simulink model "SystemArch"  (R2025a)
settings: Solver=VariableStepAuto  StartTime=0.0  StopTime=10.0  RelTol=1e-3
undefined symbols (not defined in the file): BMS, Camera, Digital, GPS, I2C, IMU, Trhemocouple, UART, UBS1, UBS2, USB1
(part 1 of 2)
settings Model: Creator=el2jo  LastModifiedBy=el2jo

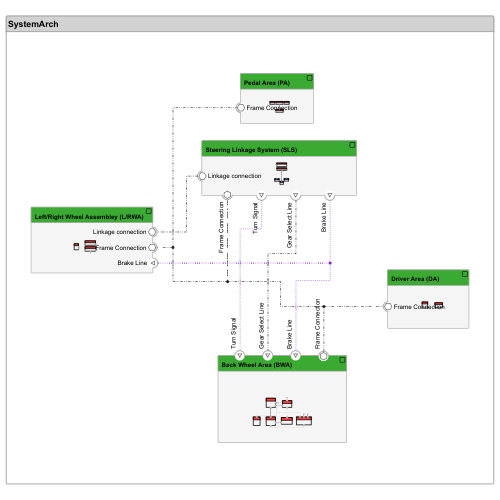
[thumbnail: Simulink's stored preview of the top-level diagram]
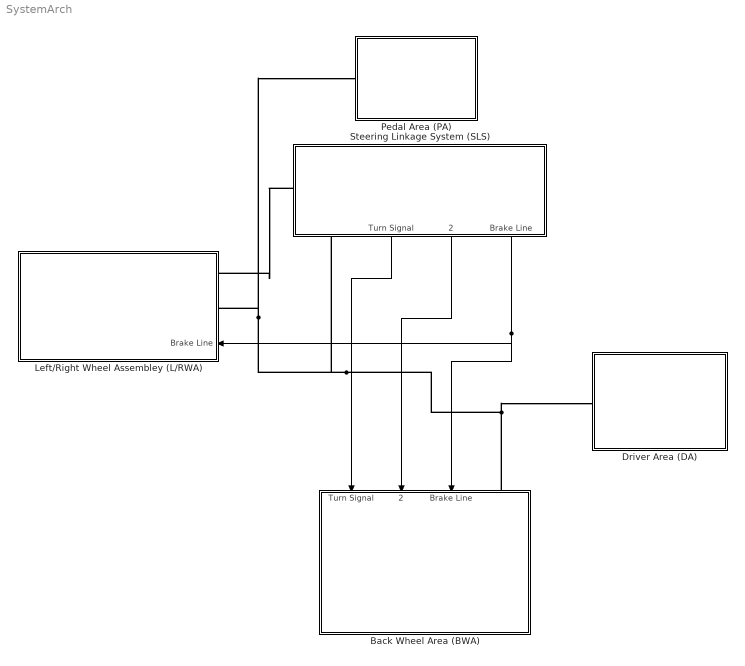
== system SystemArch ==
  "Back Wheel Area (BWA) " : Subsystem
      settings: PortSchema="{\"entries\":[{\"content\":{\"headerSize\":26,\"margin\":15,\"minimumSpacing\":25,\"sides\":[{\"content\":{},\"type\":\"ConnectorPlacement.EquallySpacedRectSide\",\"uuid\":\"b908bc96-20ac-41af-bd35-1dc4c5c5d227\"},{\"content\":{\"side\":\"RIGHT\"},\"type\":\"ConnectorPlacement.EquallySpacedRectSide\",\"uuid\":\"a58e5db6-c2cf-479b-8575-444173ed86e1\"},{\"content\":{\"connectorIds\":[\"In1\",\"In2\",\"In3\",\"LConn1\"],\"side\":\"TOP\"},\"type\":\"ConnectorPlacement.EquallySpacedRectSide\",\"uuid\":\"d8b1b400-2606-4583-b904-435fd1d8de03\"},{\"content\":{\"side\":\"BOTTOM\"},\"type\":\"ConnectorPlacement.EquallySpacedRectSide\",\"uuid\":\"75f2ceb6-2288-4f67-913e-11cbd02fad7a\"}]},\"type\":\"ConnectorPlacement.EquallySpacedConnector\",\"uuid\":\"bef962c1-e5c2-4b6f-9336-41c558e2844c\"}],\"packageUris\":[\"http://schema.mathworks.com/mf0/Connector/R2020b\"],\"version\":\"1.0\"}"
  Driver Area (DA) : Subsystem
      settings: PortSchema="{\"entries\":[{\"content\":{\"headerSize\":26,\"margin\":15,\"minimumSpacing\":25,\"sides\":[{\"content\":{\"connectorIds\":[\"RConn1\"]},\"type\":\"ConnectorPlacement.EquallySpacedRectSide\",\"uuid\":\"9a85c35e-563d-4a01-b414-04078d713158\"},{\"content\":{\"side\":\"RIGHT\"},\"type\":\"ConnectorPlacement.EquallySpacedRectSide\",\"uuid\":\"c9009d1a-5d28-4010-89bb-ea158d9a12da\"},{\"content\":{\"side\":\"TOP\"},\"type\":\"ConnectorPlacement.EquallySpacedRectSide\",\"uuid\":\"7ba794cc-3a18-4e87-89a3-ec47c4636e6e\"},{\"content\":{\"side\":\"BOTTOM\"},\"type\":\"ConnectorPlacement.EquallySpacedRectSide\",\"uuid\":\"f897e654-bc77-4131-98b6-05ede3c94ab0\"}]},\"type\":\"ConnectorPlacement.EquallySpacedConnector\",\"uuid\":\"a2b4ff38-2813-4eb8-955a-97f08d182cf4\"}],\"packageUris\":[\"http://schema.mathworks.com/mf0/Connector/R2020b\"],\"version\":\"1.0\"}"
  Left/Right Wheel Assembley (L/RWA) : Subsystem
      settings: PortSchema="{\"entries\":[{\"content\":{\"headerSize\":26,\"margin\":15,\"minimumSpacing\":25,\"sides\":[{\"content\":{},\"type\":\"ConnectorPlacement.EquallySpacedRectSide\",\"uuid\":\"9a85c35e-563d-4a01-b414-04078d713158\"},{\"content\":{\"connectorIds\":[\"RConn1\",\"RConn2\",\"In1\"],\"side\":\"RIGHT\"},\"type\":\"ConnectorPlacement.EquallySpacedRectSide\",\"uuid\":\"c9009d1a-5d28-4010-89bb-ea158d9a12da\"},{\"content\":{\"side\":\"TOP\"},\"type\":\"ConnectorPlacement.EquallySpacedRectSide\",\"uuid\":\"7ba794cc-3a18-4e87-89a3-ec47c4636e6e\"},{\"content\":{\"side\":\"BOTTOM\"},\"type\":\"ConnectorPlacement.EquallySpacedRectSide\",\"uuid\":\"b9e3f91c-afcc-4ee7-a70b-ea22bbb4204d\"}]},\"type\":\"ConnectorPlacement.EquallySpacedConnector\",\"uuid\":\"a2b4ff38-2813-4eb8-955a-97f08d182cf4\"}],\"packageUris\":[\"http://schema.mathworks.com/mf0/Connector/R2020b\"],\"version\":\"1.0\"}"
  Pedal Area (PA) : Subsystem
      settings: PortSchema="{\"entries\":[{\"content\":{\"headerSize\":26,\"margin\":15,\"minimumSpacing\":25,\"sides\":[{\"content\":{\"connectorIds\":[\"RConn1\"]},\"type\":\"ConnectorPlacement.EquallySpacedRectSide\",\"uuid\":\"9a85c35e-563d-4a01-b414-04078d713158\"},{\"content\":{\"side\":\"RIGHT\"},\"type\":\"ConnectorPlacement.EquallySpacedRectSide\",\"uuid\":\"c9009d1a-5d28-4010-89bb-ea158d9a12da\"},{\"content\":{\"side\":\"TOP\"},\"type\":\"ConnectorPlacement.EquallySpacedRectSide\",\"uuid\":\"7ba794cc-3a18-4e87-89a3-ec47c4636e6e\"},{\"content\":{\"side\":\"BOTTOM\"},\"type\":\"ConnectorPlacement.EquallySpacedRectSide\",\"uuid\":\"443625ad-4830-4e83-8594-463a9c2e837b\"}]},\"type\":\"ConnectorPlacement.EquallySpacedConnector\",\"uuid\":\"a2b4ff38-2813-4eb8-955a-97f08d182cf4\"}],\"packageUris\":[\"http://schema.mathworks.com/mf0/Connector/R2020b\"],\"version\":\"1.0\"}"
  Steering Linkage System (SLS) : Subsystem
      settings: PortSchema="{\"entries\":[{\"content\":{\"headerSize\":26,\"margin\":15,\"minimumSpacing\":25,\"sides\":[{\"content\":{\"connectorIds\":[\"RConn1\"]},\"type\":\"ConnectorPlacement.EquallySpacedRectSide\",\"uuid\":\"9a85c35e-563d-4a01-b414-04078d713158\"},{\"content\":{\"side\":\"RIGHT\"},\"type\":\"ConnectorPlacement.EquallySpacedRectSide\",\"uuid\":\"c9009d1a-5d28-4010-89bb-ea158d9a12da\"},{\"content\":{\"side\":\"TOP\"},\"type\":\"ConnectorPlacement.EquallySpacedRectSide\",\"uuid\":\"7ba794cc-3a18-4e87-89a3-ec47c4636e6e\"},{\"content\":{\"connectorIds\":[\"RConn2\",\"Out1\",\"Out2\",\"Out3\"],\"side\":\"BOTTOM\"},\"type\":\"ConnectorPlacement.EquallySpacedRectSide\",\"uuid\":\"ee526e7b-a27e-4264-aa86-39ffcd82e9f9\"}]},\"type\":\"ConnectorPlacement.EquallySpacedConnector\",\"uuid\":\"a2b4ff38-2813-4eb8-955a-97f08d182cf4\"}],\"packageUris\":[\"http://schema.mathworks.com/mf0/Connector/R2020b\"],\"version\":\"1.0\"}"
  wires:
  Steering Linkage System (SLS)/1(Turn Signal) -> "Back Wheel Area (BWA) "/1(Turn Signal)
  Steering Linkage System (SLS)/2(Gear Select Line) -> "Back Wheel Area (BWA) "/2(Gear Select Line)
  Steering Linkage System (SLS)/3(Brake Line) -> Left/Right Wheel Assembley (L/RWA)/1(Brake Line), "Back Wheel Area (BWA) "/3(Brake Line)
  connections:
  "Back Wheel Area (BWA) "/LConn1 -- Steering Linkage System (SLS)/RConn2 -- Pedal Area (PA)/RConn1 -- Left/Right Wheel Assembley (L/RWA)/RConn2 -- Driver Area (DA)/RConn1
  Steering Linkage System (SLS)/RConn1 -- Left/Right Wheel Assembley (L/RWA)/RConn1

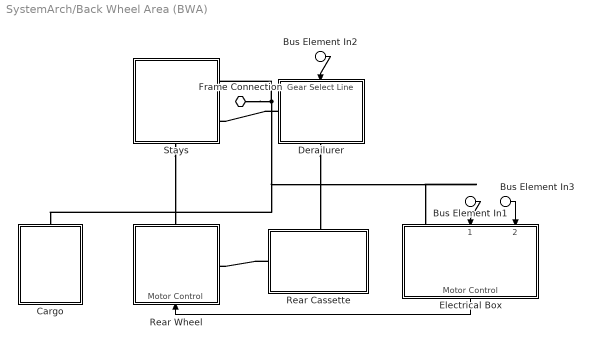
== system SystemArch/Back Wheel Area (BWA)  ==
  Bus Element In1 : Inport  PortName=Turn Signal
  Bus Element In2 : Inport  Port=2  PortName=Gear Select Line
  Bus Element In3 : Inport  Port=3  PortName=Brake Line
  "  Rear Cassette" : Subsystem
      settings: PortSchema="{\"entries\":[{\"content\":{\"headerSize\":26,\"margin\":15,\"minimumSpacing\":25,\"sides\":[{\"content\":{\"connectorIds\":[\"LConn2\"]},\"type\":\"ConnectorPlacement.EquallySpacedRectSide\",\"uuid\":\"9a85c35e-563d-4a01-b414-04078d713158\"},{\"content\":{\"side\":\"RIGHT\"},\"type\":\"ConnectorPlacement.EquallySpacedRectSide\",\"uuid\":\"c9009d1a-5d28-4010-89bb-ea158d9a12da\"},{\"content\":{\"connectorIds\":[\"LConn1\"],\"side\":\"TOP\"},\"type\":\"ConnectorPlacement.EquallySpacedRectSide\",\"uuid\":\"7ba794cc-3a18-4e87-89a3-ec47c4636e6e\"}]},\"type\":\"ConnectorPlacement.EquallySpacedConnector\",\"uuid\":\"a2b4ff38-2813-4eb8-955a-97f08d182cf4\"}],\"packageUris\":[\"http://schema.mathworks.com/mf0/Connector/R2020b\"],\"version\":\"1.0\"}"
  Cargo : Subsystem
      settings: PortSchema="{\"entries\":[{\"content\":{\"headerSize\":26,\"margin\":15,\"minimumSpacing\":25,\"sides\":[{\"content\":{},\"type\":\"ConnectorPlacement.EquallySpacedRectSide\",\"uuid\":\"9a85c35e-563d-4a01-b414-04078d713158\"},{\"content\":{\"side\":\"RIGHT\"},\"type\":\"ConnectorPlacement.EquallySpacedRectSide\",\"uuid\":\"c9009d1a-5d28-4010-89bb-ea158d9a12da\"},{\"content\":{\"connectorIds\":[\"LConn1\"],\"side\":\"TOP\"},\"type\":\"ConnectorPlacement.EquallySpacedRectSide\",\"uuid\":\"7ba794cc-3a18-4e87-89a3-ec47c4636e6e\"}]},\"type\":\"ConnectorPlacement.EquallySpacedConnector\",\"uuid\":\"a2b4ff38-2813-4eb8-955a-97f08d182cf4\"}],\"packageUris\":[\"http://schema.mathworks.com/mf0/Connector/R2020b\"],\"version\":\"1.0\"}"
  Derailurer : Subsystem
      settings: PortSchema="{\"entries\":[{\"content\":{\"headerSize\":26,\"margin\":15,\"minimumSpacing\":25,\"sides\":[{\"content\":{\"connectorIds\":[\"LConn1\"]},\"type\":\"ConnectorPlacement.EquallySpacedRectSide\",\"uuid\":\"9a85c35e-563d-4a01-b414-04078d713158\"},{\"content\":{\"side\":\"RIGHT\"},\"type\":\"ConnectorPlacement.EquallySpacedRectSide\",\"uuid\":\"c9009d1a-5d28-4010-89bb-ea158d9a12da\"},{\"content\":{\"connectorIds\":[\"In1\"],\"side\":\"TOP\"},\"type\":\"ConnectorPlacement.EquallySpacedRectSide\",\"uuid\":\"7ba794cc-3a18-4e87-89a3-ec47c4636e6e\"},{\"content\":{\"connectorIds\":[\"RConn1\"],\"side\":\"BOTTOM\"},\"type\":\"ConnectorPlacement.EquallySpacedRectSide\",\"uuid\":\"612b2382-3768-40cf-8c67-0c3e27c64c6d\"}]},\"type\":\"ConnectorPlacement.EquallySpacedConnector\",\"uuid\":\"a2b4ff38-2813-4eb8-955a-97f08d182cf4\"}],\"packageUris\":[\"http://schema.mathworks.com/mf0/Connector/R2020b\"],\"version\":\"1.0\"}"
  Electrical Box : Subsystem
      settings: PortSchema="{\"entries\":[{\"content\":{\"headerSize\":26,\"margin\":15,\"minimumSpacing\":25,\"sides\":[{\"content\":{},\"type\":\"ConnectorPlacement.EquallySpacedRectSide\",\"uuid\":\"b908bc96-20ac-41af-bd35-1dc4c5c5d227\"},{\"content\":{\"side\":\"RIGHT\"},\"type\":\"ConnectorPlacement.EquallySpacedRectSide\",\"uuid\":\"a58e5db6-c2cf-479b-8575-444173ed86e1\"},{\"content\":{\"connectorIds\":[\"LConn1\",\"In1\",\"In2\"],\"side\":\"TOP\"},\"type\":\"ConnectorPlacement.EquallySpacedRectSide\",\"uuid\":\"d8b1b400-2606-4583-b904-435fd1d8de03\"},{\"content\":{\"connectorIds\":[\"Out1\"],\"side\":\"BOTTOM\"},\"type\":\"ConnectorPlacement.EquallySpacedRectSide\",\"uuid\":\"a50bf375-f8fa-400b-8497-e942a7ca09d1\"}]},\"type\":\"ConnectorPlacement.EquallySpacedConnector\",\"uuid\":\"bef962c1-e5c2-4b6f-9336-41c558e2844c\"}],\"packageUris\":[\"http://schema.mathworks.com/mf0/Connector/R2020b\"],\"version\":\"1.0\"}"
  Rear Wheel : Subsystem
      settings: PortSchema="{\"entries\":[{\"content\":{\"headerSize\":26,\"margin\":15,\"minimumSpacing\":25,\"sides\":[{\"content\":{},\"type\":\"ConnectorPlacement.EquallySpacedRectSide\",\"uuid\":\"9a85c35e-563d-4a01-b414-04078d713158\"},{\"content\":{\"connectorIds\":[\"RConn1\"],\"side\":\"RIGHT\"},\"type\":\"ConnectorPlacement.EquallySpacedRectSide\",\"uuid\":\"c9009d1a-5d28-4010-89bb-ea158d9a12da\"},{\"content\":{\"connectorIds\":[\"LConn1\"],\"side\":\"TOP\"},\"type\":\"ConnectorPlacement.EquallySpacedRectSide\",\"uuid\":\"7ba794cc-3a18-4e87-89a3-ec47c4636e6e\"},{\"content\":{\"connectorIds\":[\"In1\"],\"side\":\"BOTTOM\"},\"type\":\"ConnectorPlacement.EquallySpacedRectSide\",\"uuid\":\"790efda8-cec0-4a27-8622-bef3d471aaff\"}]},\"type\":\"ConnectorPlacement.EquallySpacedConnector\",\"uuid\":\"a2b4ff38-2813-4eb8-955a-97f08d182cf4\"}],\"packageUris\":[\"http://schema.mathworks.com/mf0/Connector/R2020b\"],\"version\":\"1.0\"}"
  Stays : Subsystem
      settings: PortSchema="{\"entries\":[{\"content\":{\"headerSize\":26,\"margin\":15,\"minimumSpacing\":25,\"sides\":[{\"content\":{},\"type\":\"ConnectorPlacement.EquallySpacedRectSide\",\"uuid\":\"9a85c35e-563d-4a01-b414-04078d713158\"},{\"content\":{\"connectorIds\":[\"LConn1\",\"RConn1\"],\"side\":\"RIGHT\"},\"type\":\"ConnectorPlacement.EquallySpacedRectSide\",\"uuid\":\"c9009d1a-5d28-4010-89bb-ea158d9a12da\"},{\"content\":{\"side\":\"TOP\"},\"type\":\"ConnectorPlacement.EquallySpacedRectSide\",\"uuid\":\"7ba794cc-3a18-4e87-89a3-ec47c4636e6e\"},{\"content\":{\"connectorIds\":[\"RConn2\"],\"side\":\"BOTTOM\"},\"type\":\"ConnectorPlacement.EquallySpacedRectSide\",\"uuid\":\"d8ca6e35-2892-477f-b035-8e0ebcbafa05\"}]},\"type\":\"ConnectorPlacement.EquallySpacedConnector\",\"uuid\":\"a2b4ff38-2813-4eb8-955a-97f08d182cf4\"}],\"packageUris\":[\"http://schema.mathworks.com/mf0/Connector/R2020b\"],\"version\":\"1.0\"}"
  Frame Connection : PMIOPort  Side=Left
  wires:
  Electrical Box/1(Motor Control) -> Rear Wheel/1(Motor Control)
  Bus Element In2/1 -> Derailurer/1(Gear Select Line)
  Bus Element In1/1 -> Electrical Box/1(Turn Signal)
  Bus Element In3/1 -> Electrical Box/2(Brake Line)
  connections:
  Stays/RConn2 -- Rear Wheel/LConn1
  Frame Connection/RConn1 -- Cargo/LConn1 -- Electrical Box/LConn1 -- Stays/LConn1
  "  Rear Cassette"/LConn2 -- Rear Wheel/RConn1
  Derailurer/LConn1 -- Stays/RConn1
  Derailurer/RConn1 -- "  Rear Cassette"/LConn1

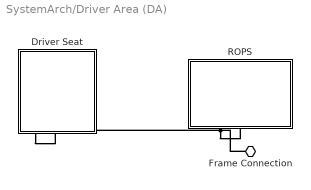
== system SystemArch/Driver Area (DA) ==
  Driver Seat : Subsystem
      settings: PortSchema="{\"entries\":[{\"content\":{\"headerSize\":26,\"margin\":15,\"minimumSpacing\":25,\"sides\":[{\"content\":{},\"type\":\"ConnectorPlacement.EquallySpacedRectSide\",\"uuid\":\"9a85c35e-563d-4a01-b414-04078d713158\"},{\"content\":{\"side\":\"RIGHT\"},\"type\":\"ConnectorPlacement.EquallySpacedRectSide\",\"uuid\":\"c9009d1a-5d28-4010-89bb-ea158d9a12da\"},{\"content\":{\"side\":\"TOP\"},\"type\":\"ConnectorPlacement.EquallySpacedRectSide\",\"uuid\":\"7ba794cc-3a18-4e87-89a3-ec47c4636e6e\"},{\"content\":{\"connectorIds\":[\"RConn1\"],\"side\":\"BOTTOM\"},\"type\":\"ConnectorPlacement.EquallySpacedRectSide\",\"uuid\":\"08e026bb-01c5-465b-bb8c-e734b87ff441\"}]},\"type\":\"ConnectorPlacement.EquallySpacedConnector\",\"uuid\":\"a2b4ff38-2813-4eb8-955a-97f08d182cf4\"}],\"packageUris\":[\"http://schema.mathworks.com/mf0/Connector/R2020b\"],\"version\":\"1.0\"}"
  ROPS : Subsystem
      settings: PortSchema="{\"entries\":[{\"content\":{\"headerSize\":26,\"margin\":15,\"minimumSpacing\":25,\"sides\":[{\"content\":{},\"type\":\"ConnectorPlacement.EquallySpacedRectSide\",\"uuid\":\"9a85c35e-563d-4a01-b414-04078d713158\"},{\"content\":{\"side\":\"RIGHT\"},\"type\":\"ConnectorPlacement.EquallySpacedRectSide\",\"uuid\":\"c9009d1a-5d28-4010-89bb-ea158d9a12da\"},{\"content\":{\"side\":\"TOP\"},\"type\":\"ConnectorPlacement.EquallySpacedRectSide\",\"uuid\":\"7ba794cc-3a18-4e87-89a3-ec47c4636e6e\"},{\"content\":{\"connectorIds\":[\"RConn1\"],\"side\":\"BOTTOM\"},\"type\":\"ConnectorPlacement.EquallySpacedRectSide\",\"uuid\":\"f6e8be95-bb09-4692-bbab-764924998958\"}]},\"type\":\"ConnectorPlacement.EquallySpacedConnector\",\"uuid\":\"a2b4ff38-2813-4eb8-955a-97f08d182cf4\"}],\"packageUris\":[\"http://schema.mathworks.com/mf0/Connector/R2020b\"],\"version\":\"1.0\"}"
  Frame Connection : PMIOPort  Side=Right
  connections:
  Frame Connection/RConn1 -- Driver Seat/RConn1 -- ROPS/RConn1

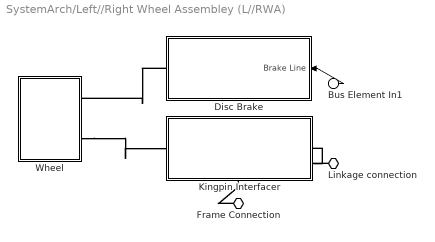
== system SystemArch/Left//Right Wheel Assembley (L//RWA) ==
  Bus Element In1 : Inport  PortName=Brake Line
  Disc Brake : Subsystem
      settings: PortSchema="{\"entries\":[{\"content\":{\"headerSize\":26,\"margin\":15,\"minimumSpacing\":25,\"sides\":[{\"content\":{\"connectorIds\":[\"LConn1\"]},\"type\":\"ConnectorPlacement.EquallySpacedRectSide\",\"uuid\":\"9a85c35e-563d-4a01-b414-04078d713158\"},{\"content\":{\"connectorIds\":[\"In1\"],\"side\":\"RIGHT\"},\"type\":\"ConnectorPlacement.EquallySpacedRectSide\",\"uuid\":\"c9009d1a-5d28-4010-89bb-ea158d9a12da\"},{\"content\":{\"side\":\"TOP\"},\"type\":\"ConnectorPlacement.EquallySpacedRectSide\",\"uuid\":\"7ba794cc-3a18-4e87-89a3-ec47c4636e6e\"}]},\"type\":\"ConnectorPlacement.EquallySpacedConnector\",\"uuid\":\"a2b4ff38-2813-4eb8-955a-97f08d182cf4\"}],\"packageUris\":[\"http://schema.mathworks.com/mf0/Connector/R2020b\"],\"version\":\"1.0\"}"
  Kingpin Interfacer : Subsystem
      settings: PortSchema="{\"entries\":[{\"content\":{\"headerSize\":26,\"margin\":15,\"minimumSpacing\":25,\"sides\":[{\"content\":{\"connectorIds\":[\"RConn3\"]},\"type\":\"ConnectorPlacement.EquallySpacedRectSide\",\"uuid\":\"9a85c35e-563d-4a01-b414-04078d713158\"},{\"content\":{\"connectorIds\":[\"RConn2\"],\"side\":\"RIGHT\"},\"type\":\"ConnectorPlacement.EquallySpacedRectSide\",\"uuid\":\"c9009d1a-5d28-4010-89bb-ea158d9a12da\"},{\"content\":{\"side\":\"TOP\"},\"type\":\"ConnectorPlacement.EquallySpacedRectSide\",\"uuid\":\"7ba794cc-3a18-4e87-89a3-ec47c4636e6e\"},{\"content\":{\"connectorIds\":[\"RConn1\"],\"side\":\"BOTTOM\"},\"type\":\"ConnectorPlacement.EquallySpacedRectSide\",\"uuid\":\"1146683b-fd7d-4bc2-bfc7-5416f68f0a28\"}]},\"type\":\"ConnectorPlacement.EquallySpacedConnector\",\"uuid\":\"a2b4ff38-2813-4eb8-955a-97f08d182cf4\"}],\"packageUris\":[\"http://schema.mathworks.com/mf0/Connector/R2020b\"],\"version\":\"1.0\"}"
  Wheel : Subsystem
      settings: PortSchema="{\"entries\":[{\"content\":{\"headerSize\":26,\"margin\":15,\"minimumSpacing\":25,\"sides\":[{\"content\":{},\"type\":\"ConnectorPlacement.EquallySpacedRectSide\",\"uuid\":\"9a85c35e-563d-4a01-b414-04078d713158\"},{\"content\":{\"connectorIds\":[\"RConn1\",\"RConn2\"],\"side\":\"RIGHT\"},\"type\":\"ConnectorPlacement.EquallySpacedRectSide\",\"uuid\":\"c9009d1a-5d28-4010-89bb-ea158d9a12da\"},{\"content\":{\"side\":\"TOP\"},\"type\":\"ConnectorPlacement.EquallySpacedRectSide\",\"uuid\":\"7ba794cc-3a18-4e87-89a3-ec47c4636e6e\"},{\"content\":{\"side\":\"BOTTOM\"},\"type\":\"ConnectorPlacement.EquallySpacedRectSide\",\"uuid\":\"b840c23f-69d1-4217-b707-91eb7d19865c\"}]},\"type\":\"ConnectorPlacement.EquallySpacedConnector\",\"uuid\":\"a2b4ff38-2813-4eb8-955a-97f08d182cf4\"}],\"packageUris\":[\"http://schema.mathworks.com/mf0/Connector/R2020b\"],\"version\":\"1.0\"}"
  Linkage connection : PMIOPort  Side=Right
  Frame Connection : PMIOPort  Port=2  Side=Right
  wires:
  Bus Element In1/1 -> Disc Brake/1(Brake Line)
  connections:
  Wheel/RConn2 -- Kingpin Interfacer/RConn3
  Disc Brake/LConn1 -- Wheel/RConn1
  Linkage connection/RConn1 -- Kingpin Interfacer/RConn2
  Frame Connection/RConn1 -- Kingpin Interfacer/RConn1

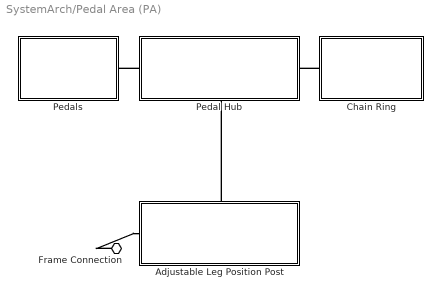
== system SystemArch/Pedal Area (PA) ==
  Adjustable Leg Position Post : Subsystem
      settings: PortSchema="{\"entries\":[{\"content\":{\"headerSize\":26,\"margin\":15,\"minimumSpacing\":25,\"sides\":[{\"content\":{\"connectorIds\":[\"LConn1\"]},\"type\":\"ConnectorPlacement.EquallySpacedRectSide\",\"uuid\":\"9a85c35e-563d-4a01-b414-04078d713158\"},{\"content\":{\"side\":\"RIGHT\"},\"type\":\"ConnectorPlacement.EquallySpacedRectSide\",\"uuid\":\"c9009d1a-5d28-4010-89bb-ea158d9a12da\"},{\"content\":{\"connectorIds\":[\"LConn2\"],\"side\":\"TOP\"},\"type\":\"ConnectorPlacement.EquallySpacedRectSide\",\"uuid\":\"7ba794cc-3a18-4e87-89a3-ec47c4636e6e\"}]},\"type\":\"ConnectorPlacement.EquallySpacedConnector\",\"uuid\":\"a2b4ff38-2813-4eb8-955a-97f08d182cf4\"}],\"packageUris\":[\"http://schema.mathworks.com/mf0/Connector/R2020b\"],\"version\":\"1.0\"}"
  Chain Ring : Subsystem
      settings: PortSchema="{\"entries\":[{\"content\":{\"headerSize\":26,\"margin\":15,\"minimumSpacing\":25,\"sides\":[{\"content\":{\"connectorIds\":[\"LConn1\"]},\"type\":\"ConnectorPlacement.EquallySpacedRectSide\",\"uuid\":\"9a85c35e-563d-4a01-b414-04078d713158\"},{\"content\":{\"side\":\"RIGHT\"},\"type\":\"ConnectorPlacement.EquallySpacedRectSide\",\"uuid\":\"c9009d1a-5d28-4010-89bb-ea158d9a12da\"},{\"content\":{\"side\":\"TOP\"},\"type\":\"ConnectorPlacement.EquallySpacedRectSide\",\"uuid\":\"7ba794cc-3a18-4e87-89a3-ec47c4636e6e\"}]},\"type\":\"ConnectorPlacement.EquallySpacedConnector\",\"uuid\":\"a2b4ff38-2813-4eb8-955a-97f08d182cf4\"}],\"packageUris\":[\"http://schema.mathworks.com/mf0/Connector/R2020b\"],\"version\":\"1.0\"}"
  Pedal Hub : Subsystem
      settings: PortSchema="{\"entries\":[{\"content\":{\"headerSize\":26,\"margin\":15,\"minimumSpacing\":25,\"sides\":[{\"content\":{\"connectorIds\":[\"LConn1\"]},\"type\":\"ConnectorPlacement.EquallySpacedRectSide\",\"uuid\":\"9a85c35e-563d-4a01-b414-04078d713158\"},{\"content\":{\"connectorIds\":[\"RConn1\"],\"side\":\"RIGHT\"},\"type\":\"ConnectorPlacement.EquallySpacedRectSide\",\"uuid\":\"c9009d1a-5d28-4010-89bb-ea158d9a12da\"},{\"content\":{\"side\":\"TOP\"},\"type\":\"ConnectorPlacement.EquallySpacedRectSide\",\"uuid\":\"7ba794cc-3a18-4e87-89a3-ec47c4636e6e\"},{\"content\":{\"connectorIds\":[\"RConn2\"],\"side\":\"BOTTOM\"},\"type\":\"ConnectorPlacement.EquallySpacedRectSide\",\"uuid\":\"d446abce-ebed-4a7d-b07b-7c209b5faf41\"}]},\"type\":\"ConnectorPlacement.EquallySpacedConnector\",\"uuid\":\"a2b4ff38-2813-4eb8-955a-97f08d182cf4\"}],\"packageUris\":[\"http://schema.mathworks.com/mf0/Connector/R2020b\"],\"version\":\"1.0\"}"
  Pedals : Subsystem
      settings: PortSchema="{\"entries\":[{\"content\":{\"headerSize\":26,\"margin\":15,\"minimumSpacing\":25,\"sides\":[{\"content\":{},\"type\":\"ConnectorPlacement.EquallySpacedRectSide\",\"uuid\":\"9a85c35e-563d-4a01-b414-04078d713158\"},{\"content\":{\"connectorIds\":[\"RConn1\"],\"side\":\"RIGHT\"},\"type\":\"ConnectorPlacement.EquallySpacedRectSide\",\"uuid\":\"c9009d1a-5d28-4010-89bb-ea158d9a12da\"},{\"content\":{\"side\":\"TOP\"},\"type\":\"ConnectorPlacement.EquallySpacedRectSide\",\"uuid\":\"7ba794cc-3a18-4e87-89a3-ec47c4636e6e\"}]},\"type\":\"ConnectorPlacement.EquallySpacedConnector\",\"uuid\":\"a2b4ff38-2813-4eb8-955a-97f08d182cf4\"}],\"packageUris\":[\"http://schema.mathworks.com/mf0/Connector/R2020b\"],\"version\":\"1.0\"}"
  Frame Connection : PMIOPort  Side=Right
  connections:
  Adjustable Leg Position Post/LConn2 -- Pedal Hub/RConn2
  Frame Connection/RConn1 -- Adjustable Leg Position Post/LConn1
  Chain Ring/LConn1 -- Pedal Hub/RConn1
  Pedal Hub/LConn1 -- Pedals/RConn1

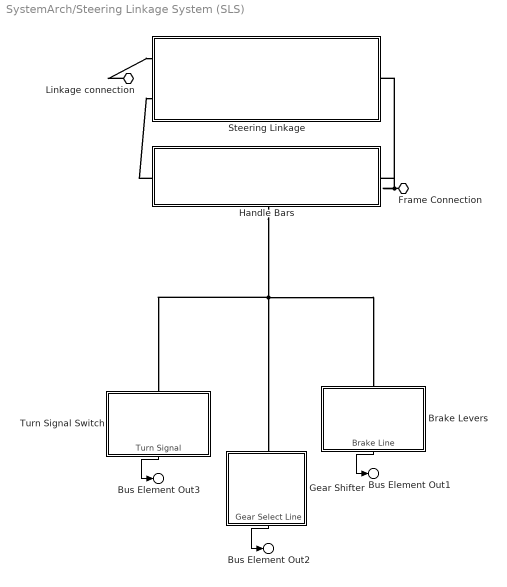
== system SystemArch/Steering Linkage System (SLS) ==
  Brake Levers : Subsystem
      settings: PortSchema="{\"entries\":[{\"content\":{\"headerSize\":26,\"margin\":15,\"minimumSpacing\":25,\"sides\":[{\"content\":{},\"type\":\"ConnectorPlacement.EquallySpacedRectSide\",\"uuid\":\"9a85c35e-563d-4a01-b414-04078d713158\"},{\"content\":{\"side\":\"RIGHT\"},\"type\":\"ConnectorPlacement.EquallySpacedRectSide\",\"uuid\":\"c9009d1a-5d28-4010-89bb-ea158d9a12da\"},{\"content\":{\"connectorIds\":[\"LConn1\"],\"side\":\"TOP\"},\"type\":\"ConnectorPlacement.EquallySpacedRectSide\",\"uuid\":\"7ba794cc-3a18-4e87-89a3-ec47c4636e6e\"},{\"content\":{\"connectorIds\":[\"Out1\"],\"side\":\"BOTTOM\"},\"type\":\"ConnectorPlacement.EquallySpacedRectSide\",\"uuid\":\"d36662b7-eafd-4fe1-9f34-893244a16a70\"}]},\"type\":\"ConnectorPlacement.EquallySpacedConnector\",\"uuid\":\"a2b4ff38-2813-4eb8-955a-97f08d182cf4\"}],\"packageUris\":[\"http://schema.mathworks.com/mf0/Connector/R2020b\"],\"version\":\"1.0\"}"
  Gear Shifter : Subsystem
      settings: PortSchema="{\"entries\":[{\"content\":{\"headerSize\":26,\"margin\":15,\"minimumSpacing\":25,\"sides\":[{\"content\":{},\"type\":\"ConnectorPlacement.EquallySpacedRectSide\",\"uuid\":\"9a85c35e-563d-4a01-b414-04078d713158\"},{\"content\":{\"side\":\"RIGHT\"},\"type\":\"ConnectorPlacement.EquallySpacedRectSide\",\"uuid\":\"c9009d1a-5d28-4010-89bb-ea158d9a12da\"},{\"content\":{\"connectorIds\":[\"LConn1\"],\"side\":\"TOP\"},\"type\":\"ConnectorPlacement.EquallySpacedRectSide\",\"uuid\":\"7ba794cc-3a18-4e87-89a3-ec47c4636e6e\"},{\"content\":{\"connectorIds\":[\"Out1\"],\"side\":\"BOTTOM\"},\"type\":\"ConnectorPlacement.EquallySpacedRectSide\",\"uuid\":\"cca68fd4-9db3-4130-b142-cf5b0259fadd\"}]},\"type\":\"ConnectorPlacement.EquallySpacedConnector\",\"uuid\":\"a2b4ff38-2813-4eb8-955a-97f08d182cf4\"}],\"packageUris\":[\"http://schema.mathworks.com/mf0/Connector/R2020b\"],\"version\":\"1.0\"}"
  Handle Bars : Subsystem
      settings: PortSchema="{\"entries\":[{\"content\":{\"headerSize\":26,\"margin\":15,\"minimumSpacing\":25,\"sides\":[{\"content\":{\"connectorIds\":[\"LConn1\"]},\"type\":\"ConnectorPlacement.EquallySpacedRectSide\",\"uuid\":\"9a85c35e-563d-4a01-b414-04078d713158\"},{\"content\":{\"connectorIds\":[\"RConn2\"],\"side\":\"RIGHT\"},\"type\":\"ConnectorPlacement.EquallySpacedRectSide\",\"uuid\":\"c9009d1a-5d28-4010-89bb-ea158d9a12da\"},{\"content\":{\"side\":\"TOP\"},\"type\":\"ConnectorPlacement.EquallySpacedRectSide\",\"uuid\":\"7ba794cc-3a18-4e87-89a3-ec47c4636e6e\"},{\"content\":{\"connectorIds\":[\"RConn1\"],\"side\":\"BOTTOM\"},\"type\":\"ConnectorPlacement.EquallySpacedRectSide\",\"uuid\":\"88f565ff-a4ca-49c0-967e-ff026cea0d9c\"}]},\"type\":\"ConnectorPlacement.EquallySpacedConnector\",\"uuid\":\"a2b4ff38-2813-4eb8-955a-97f08d182cf4\"}],\"packageUris\":[\"http://schema.mathworks.com/mf0/Connector/R2020b\"],\"version\":\"1.0\"}"
  Steering Linkage : Subsystem
      settings: PortSchema="{\"entries\":[{\"content\":{\"headerSize\":26,\"margin\":15,\"minimumSpacing\":25,\"sides\":[{\"content\":{\"connectorIds\":[\"LConn1\",\"RConn2\"]},\"type\":\"ConnectorPlacement.EquallySpacedRectSide\",\"uuid\":\"9a85c35e-563d-4a01-b414-04078d713158\"},{\"content\":{\"connectorIds\":[\"RConn1\"],\"side\":\"RIGHT\"},\"type\":\"ConnectorPlacement.EquallySpacedRectSide\",\"uuid\":\"c9009d1a-5d28-4010-89bb-ea158d9a12da\"},{\"content\":{\"side\":\"TOP\"},\"type\":\"ConnectorPlacement.EquallySpacedRectSide\",\"uuid\":\"7ba794cc-3a18-4e87-89a3-ec47c4636e6e\"},{\"content\":{\"side\":\"BOTTOM\"},\"type\":\"ConnectorPlacement.EquallySpacedRectSide\",\"uuid\":\"26f61666-8797-4ea6-ad48-6e3ed83f096b\"}]},\"type\":\"ConnectorPlacement.EquallySpacedConnector\",\"uuid\":\"a2b4ff38-2813-4eb8-955a-97f08d182cf4\"}],\"packageUris\":[\"http://schema.mathworks.com/mf0/Connector/R2020b\"],\"version\":\"1.0\"}"
  Turn Signal Switch : Subsystem
      settings: PortSchema="{\"entries\":[{\"content\":{\"headerSize\":26,\"margin\":15,\"minimumSpacing\":25,\"sides\":[{\"content\":{},\"type\":\"ConnectorPlacement.EquallySpacedRectSide\",\"uuid\":\"9a85c35e-563d-4a01-b414-04078d713158\"},{\"content\":{\"side\":\"RIGHT\"},\"type\":\"ConnectorPlacement.EquallySpacedRectSide\",\"uuid\":\"c9009d1a-5d28-4010-89bb-ea158d9a12da\"},{\"content\":{\"connectorIds\":[\"LConn1\"],\"side\":\"TOP\"},\"type\":\"ConnectorPlacement.EquallySpacedRectSide\",\"uuid\":\"7ba794cc-3a18-4e87-89a3-ec47c4636e6e\"},{\"content\":{\"connectorIds\":[\"Out1\"],\"side\":\"BOTTOM\"},\"type\":\"ConnectorPlacement.EquallySpacedRectSide\",\"uuid\":\"83f4b132-e8e5-488d-b469-fef27ef88e02\"}]},\"type\":\"ConnectorPlacement.EquallySpacedConnector\",\"uuid\":\"a2b4ff38-2813-4eb8-955a-97f08d182cf4\"}],\"packageUris\":[\"http://schema.mathworks.com/mf0/Connector/R2020b\"],\"version\":\"1.0\"}"
  Linkage connection : PMIOPort  Side=Right
  Frame Connection : PMIOPort  Port=2  Side=Right
  Bus Element Out3 : Outport  PortName=Turn Signal
  Bus Element Out2 : Outport  Port=2  PortName=Gear Select Line
  Bus Element Out1 : Outport  Port=3  PortName=Brake Line
  wires:
  Brake Levers/1(Brake Line) -> Bus Element Out1/1
  Gear Shifter/1(Gear Select Line) -> Bus Element Out2/1
  Turn Signal Switch/1(Turn Signal) -> Bus Element Out3/1
  connections:
  Handle Bars/LConn1 -- Steering Linkage/RConn2
  Linkage connection/RConn1 -- Steering Linkage/LConn1
  Frame Connection/RConn1 -- Steering Linkage/RConn1 -- Handle Bars/RConn2
  Handle Bars/RConn1 -- Turn Signal Switch/LConn1 -- Brake Levers/LConn1 -- Gear Shifter/LConn1

== system SystemArch/Back Wheel Area (BWA) /  Rear Cassette ==
  Conn2 : PMIOPort  Side=Left
  Conn1 : PMIOPort  Port=2  Side=Left

== system SystemArch/Back Wheel Area (BWA) /Cargo ==
  Frame Connection : PMIOPort  Side=Left

== system SystemArch/Back Wheel Area (BWA) /Derailurer ==
  Bus Element In1 : Inport  PortName=Gear Select Line
  Conn1 : PMIOPort  Side=Left
  Conn2 : PMIOPort  Port=2  Side=Right

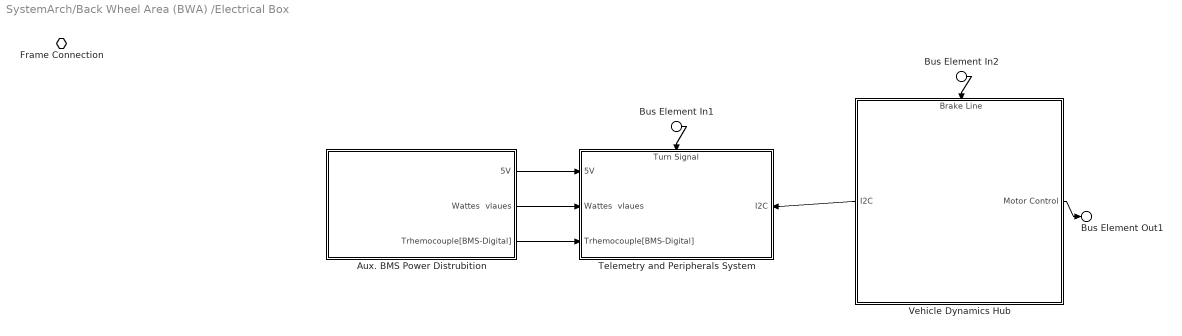
== system SystemArch/Back Wheel Area (BWA) /Electrical Box ==
  Bus Element In1 : Inport  PortName=Turn Signal
  Bus Element In2 : Inport  Port=2  PortName=Brake Line
  Aux. BMS Power Distrubition : Subsystem
      settings: PortSchema="{\"entries\":[{\"content\":{\"headerSize\":26,\"margin\":15,\"minimumSpacing\":25,\"sides\":[{\"content\":{},\"type\":\"ConnectorPlacement.EquallySpacedRectSide\",\"uuid\":\"b908bc96-20ac-41af-bd35-1dc4c5c5d227\"},{\"content\":{\"connectorIds\":[\"Out1\",\"Out2\",\"Out3\"],\"side\":\"RIGHT\"},\"type\":\"ConnectorPlacement.EquallySpacedRectSide\",\"uuid\":\"a58e5db6-c2cf-479b-8575-444173ed86e1\"},{\"content\":{\"side\":\"TOP\"},\"type\":\"ConnectorPlacement.EquallySpacedRectSide\",\"uuid\":\"d8b1b400-2606-4583-b904-435fd1d8de03\"}]},\"type\":\"ConnectorPlacement.EquallySpacedConnector\",\"uuid\":\"bef962c1-e5c2-4b6f-9336-41c558e2844c\"}],\"packageUris\":[\"http://schema.mathworks.com/mf0/Connector/R2020b\"],\"version\":\"1.0\"}"
  Telemetry and Peripherals System : Subsystem
      settings: PortSchema="{\"entries\":[{\"content\":{\"headerSize\":26,\"margin\":15,\"minimumSpacing\":25,\"sides\":[{\"content\":{\"connectorIds\":[\"In4\",\"In1\",\"In2\"]},\"type\":\"ConnectorPlacement.EquallySpacedRectSide\",\"uuid\":\"934e9821-6dd8-4ade-a7ee-3b6987477e22\"},{\"content\":{\"connectorIds\":[\"In5\"],\"side\":\"RIGHT\"},\"type\":\"ConnectorPlacement.EquallySpacedRectSide\",\"uuid\":\"f61335fe-7c5e-448a-8aa6-bab86e4b2377\"},{\"content\":{\"connectorIds\":[\"In3\"],\"side\":\"TOP\"},\"type\":\"ConnectorPlacement.EquallySpacedRectSide\",\"uuid\":\"ca2ad9c5-fde3-4c08-8e7d-48d69bab8ab0\"},{\"content\":{\"side\":\"BOTTOM\"},\"type\":\"ConnectorPlacement.EquallySpacedRectSide\",\"uuid\":\"70eac739-51a2-4044-8816-e3865dce13f0\"}]},\"type\":\"ConnectorPlacement.EquallySpacedConnector\",\"uuid\":\"1eee8468-151c-4fd8-ba6b-e50571f5f52c\"}],\"packageUris\":[\"http://schema.mathworks.com/mf0/Connector/R2020b\"],\"version\":\"1.0\"}"
  Vehicle Dynamics Hub : Subsystem
      settings: PortSchema="{\"entries\":[{\"content\":{\"headerSize\":26,\"margin\":15,\"minimumSpacing\":25,\"sides\":[{\"content\":{\"connectorIds\":[\"Out2\"]},\"type\":\"ConnectorPlacement.EquallySpacedRectSide\",\"uuid\":\"130811b4-e32d-41d0-b322-e8fa04594c75\"},{\"content\":{\"connectorIds\":[\"Out1\"],\"side\":\"RIGHT\"},\"type\":\"ConnectorPlacement.EquallySpacedRectSide\",\"uuid\":\"8119c0ce-9166-49a4-a650-142de91b8b5d\"},{\"content\":{\"connectorIds\":[\"In1\"],\"side\":\"TOP\"},\"type\":\"ConnectorPlacement.EquallySpacedRectSide\",\"uuid\":\"56beef33-baf0-4fed-91da-fc4366475bc4\"}]},\"type\":\"ConnectorPlacement.EquallySpacedConnector\",\"uuid\":\"707b8a6a-abc4-4990-9488-625113039630\"}],\"packageUris\":[\"http://schema.mathworks.com/mf0/Connector/R2020b\"],\"version\":\"1.0\"}"
  Frame Connection : PMIOPort  Side=Left
  Bus Element Out1 : Outport  PortName=Motor Control
  wires:
  Aux. BMS Power Distrubition/1(5V) -> Telemetry and Peripherals System/4(5V)
  Vehicle Dynamics Hub/2(I2C) -> Telemetry and Peripherals System/5(I2C)
  Vehicle Dynamics Hub/1(Motor Control) -> Bus Element Out1/1
  Bus Element In2/1 -> Vehicle Dynamics Hub/1(Brake Line)
  Bus Element In1/1 -> Telemetry and Peripherals System/3(Turn Signal)
  Aux. BMS Power Distrubition/3(Trhemocouple[BMS-Digital]) -> Telemetry and Peripherals System/2(Trhemocouple[BMS-Digital])
  Aux. BMS Power Distrubition/2("Wattes  vlaues ") -> Telemetry and Peripherals System/1("Wattes  vlaues ")

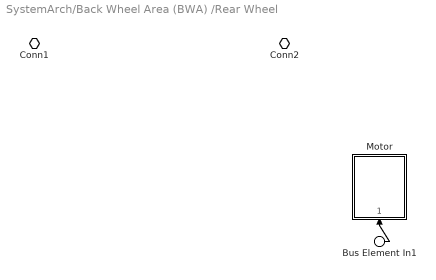
== system SystemArch/Back Wheel Area (BWA) /Rear Wheel ==
  Bus Element In1 : Inport  PortName=Motor Control
  Motor : Subsystem
      settings: PortSchema="{\"entries\":[{\"content\":{\"headerSize\":26,\"margin\":15,\"minimumSpacing\":25,\"sides\":[{\"content\":{},\"type\":\"ConnectorPlacement.EquallySpacedRectSide\",\"uuid\":\"9a85c35e-563d-4a01-b414-04078d713158\"},{\"content\":{\"side\":\"RIGHT\"},\"type\":\"ConnectorPlacement.EquallySpacedRectSide\",\"uuid\":\"c9009d1a-5d28-4010-89bb-ea158d9a12da\"},{\"content\":{\"side\":\"TOP\"},\"type\":\"ConnectorPlacement.EquallySpacedRectSide\",\"uuid\":\"7ba794cc-3a18-4e87-89a3-ec47c4636e6e\"},{\"content\":{\"connectorIds\":[\"In1\"],\"side\":\"BOTTOM\"},\"type\":\"ConnectorPlacement.EquallySpacedRectSide\",\"uuid\":\"986ce807-e5c1-4833-bcb9-c31c34acc656\"}]},\"type\":\"ConnectorPlacement.EquallySpacedConnector\",\"uuid\":\"a2b4ff38-2813-4eb8-955a-97f08d182cf4\"}],\"packageUris\":[\"http://schema.mathworks.com/mf0/Connector/R2020b\"],\"version\":\"1.0\"}"
  Conn1 : PMIOPort  Side=Left
  Conn2 : PMIOPort  Port=2  Side=Right
  wires:
  Bus Element In1/1 -> Motor/1(Motor Control)

== system SystemArch/Back Wheel Area (BWA) /Stays ==
  Conn2 : PMIOPort  Side=Right
  Conn1 : PMIOPort  Port=2  Side=Right
  Frame Connection : PMIOPort  Port=3  Side=Left

== system SystemArch/Driver Area (DA)/Driver Seat ==
  Frame Connection : PMIOPort  Side=Right

== system SystemArch/Driver Area (DA)/ROPS ==
  Frame Connection : PMIOPort  Side=Right

== system SystemArch/Left//Right Wheel Assembley (L//RWA)/Disc Brake ==
  Bus Element In1 : Inport  PortName=Brake Line
  Conn1 : PMIOPort  Side=Left

== system SystemArch/Left//Right Wheel Assembley (L//RWA)/Kingpin Interfacer ==
  Frame Connection : PMIOPort  Side=Right
  Linkage connection : PMIOPort  Port=2  Side=Right
  Conn1 : PMIOPort  Port=3  Side=Right

== system SystemArch/Left//Right Wheel Assembley (L//RWA)/Wheel ==
  Conn2 : PMIOPort  Side=Right
  Conn1 : PMIOPort  Port=2  Side=Right

== system SystemArch/Pedal Area (PA)/Adjustable Leg Position Post ==
  Frame Connection : PMIOPort  Side=Left
  Conn1 : PMIOPort  Port=2  Side=Left

== system SystemArch/Pedal Area (PA)/Chain Ring ==
  Conn1 : PMIOPort  Side=Left

== system SystemArch/Pedal Area (PA)/Pedal Hub ==
  Conn2 : PMIOPort  Side=Right
  Conn1 : PMIOPort  Port=2  Side=Right
  Conn3 : PMIOPort  Port=3  Side=Left

== system SystemArch/Pedal Area (PA)/Pedals ==
  Conn1 : PMIOPort  Side=Right

== system SystemArch/Steering Linkage System (SLS)/Brake Levers ==
  Bolted Wrap Mounting : PMIOPort  Side=Left
  Bus Element Out1 : Outport  PortName=Brake Line

== system SystemArch/Steering Linkage System (SLS)/Gear Shifter ==
  Bolted Wrap Mounting : PMIOPort  Side=Left
  Bus Element Out1 : Outport  PortName=Gear Select Line

== system SystemArch/Steering Linkage System (SLS)/Handle Bars ==
  Linkage Driver : PMIOPort  Side=Left
  Bolted Wrap Mounting : PMIOPort  Port=2  Side=Right
  Frame Connection : PMIOPort  Port=3  Side=Right

== system SystemArch/Steering Linkage System (SLS)/Steering Linkage ==
  Frame Connection : PMIOPort  Side=Right
  Linkage Driver : PMIOPort  Port=2  Side=Right
  Linkage connection : PMIOPort  Port=3  Side=Left

== system SystemArch/Steering Linkage System (SLS)/Turn Signal Switch ==
  Bolted Wrap Mounting : PMIOPort  Side=Left
  Bus Element Out1 : Outport  PortName=Turn Signal

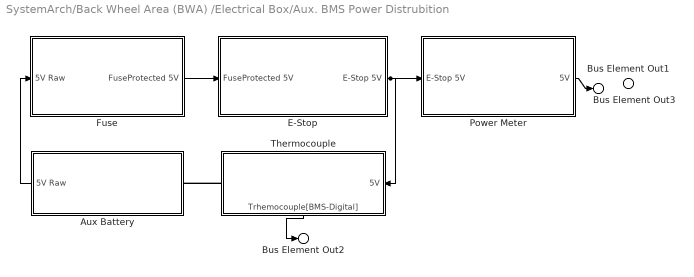
== system SystemArch/Back Wheel Area (BWA) /Electrical Box/Aux. BMS Power Distrubition ==
  Aux Battery : Subsystem
      settings: PortSchema="{\"entries\":[{\"content\":{\"headerSize\":26,\"margin\":15,\"minimumSpacing\":25,\"sides\":[{\"content\":{\"connectorIds\":[\"Out1\"]},\"type\":\"ConnectorPlacement.EquallySpacedRectSide\",\"uuid\":\"b908bc96-20ac-41af-bd35-1dc4c5c5d227\"},{\"content\":{\"connectorIds\":[\"RConn1\"],\"side\":\"RIGHT\"},\"type\":\"ConnectorPlacement.EquallySpacedRectSide\",\"uuid\":\"a58e5db6-c2cf-479b-8575-444173ed86e1\"},{\"content\":{\"side\":\"TOP\"},\"type\":\"ConnectorPlacement.EquallySpacedRectSide\",\"uuid\":\"d8b1b400-2606-4583-b904-435fd1d8de03\"}]},\"type\":\"ConnectorPlacement.EquallySpacedConnector\",\"uuid\":\"bef962c1-e5c2-4b6f-9336-41c558e2844c\"}],\"packageUris\":[\"http://schema.mathworks.com/mf0/Connector/R2020b\"],\"version\":\"1.0\"}"
  E-Stop : Subsystem
      settings: PortSchema="{\"entries\":[{\"content\":{\"headerSize\":26,\"margin\":15,\"minimumSpacing\":25,\"sides\":[{\"content\":{\"connectorIds\":[\"In1\"]},\"type\":\"ConnectorPlacement.EquallySpacedRectSide\",\"uuid\":\"b908bc96-20ac-41af-bd35-1dc4c5c5d227\"},{\"content\":{\"connectorIds\":[\"Out1\"],\"side\":\"RIGHT\"},\"type\":\"ConnectorPlacement.EquallySpacedRectSide\",\"uuid\":\"a58e5db6-c2cf-479b-8575-444173ed86e1\"},{\"content\":{\"side\":\"TOP\"},\"type\":\"ConnectorPlacement.EquallySpacedRectSide\",\"uuid\":\"d8b1b400-2606-4583-b904-435fd1d8de03\"}]},\"type\":\"ConnectorPlacement.EquallySpacedConnector\",\"uuid\":\"bef962c1-e5c2-4b6f-9336-41c558e2844c\"}],\"packageUris\":[\"http://schema.mathworks.com/mf0/Connector/R2020b\"],\"version\":\"1.0\"}"
  Fuse : Subsystem
      settings: PortSchema="{\"entries\":[{\"content\":{\"headerSize\":26,\"margin\":15,\"minimumSpacing\":25,\"sides\":[{\"content\":{\"connectorIds\":[\"In1\"]},\"type\":\"ConnectorPlacement.EquallySpacedRectSide\",\"uuid\":\"b908bc96-20ac-41af-bd35-1dc4c5c5d227\"},{\"content\":{\"connectorIds\":[\"Out1\"],\"side\":\"RIGHT\"},\"type\":\"ConnectorPlacement.EquallySpacedRectSide\",\"uuid\":\"a58e5db6-c2cf-479b-8575-444173ed86e1\"},{\"content\":{\"side\":\"TOP\"},\"type\":\"ConnectorPlacement.EquallySpacedRectSide\",\"uuid\":\"d8b1b400-2606-4583-b904-435fd1d8de03\"}]},\"type\":\"ConnectorPlacement.EquallySpacedConnector\",\"uuid\":\"bef962c1-e5c2-4b6f-9336-41c558e2844c\"}],\"packageUris\":[\"http://schema.mathworks.com/mf0/Connector/R2020b\"],\"version\":\"1.0\"}"
  Power Meter : Subsystem
      settings: PortSchema="{\"entries\":[{\"content\":{\"headerSize\":26,\"margin\":15,\"minimumSpacing\":25,\"sides\":[{\"content\":{\"connectorIds\":[\"In1\"]},\"type\":\"ConnectorPlacement.EquallySpacedRectSide\",\"uuid\":\"e53759f5-b690-4877-b44a-d4eac11dffdb\"},{\"content\":{\"connectorIds\":[\"Out1\"],\"side\":\"RIGHT\"},\"type\":\"ConnectorPlacement.EquallySpacedRectSide\",\"uuid\":\"5814382e-6b7a-453f-be59-81d6220d088b\"},{\"content\":{\"side\":\"TOP\"},\"type\":\"ConnectorPlacement.EquallySpacedRectSide\",\"uuid\":\"b6b1eca2-b862-4844-b743-dac7054e5132\"}]},\"type\":\"ConnectorPlacement.EquallySpacedConnector\",\"uuid\":\"c2feee16-aff2-42ba-93bb-380b1af0aee9\"}],\"packageUris\":[\"http://schema.mathworks.com/mf0/Connector/R2020b\"],\"version\":\"1.0\"}"
  Thermocouple : Subsystem
      settings: PortSchema="{\"entries\":[{\"content\":{\"headerSize\":26,\"margin\":15,\"minimumSpacing\":25,\"sides\":[{\"content\":{\"connectorIds\":[\"RConn1\"]},\"type\":\"ConnectorPlacement.EquallySpacedRectSide\",\"uuid\":\"b908bc96-20ac-41af-bd35-1dc4c5c5d227\"},{\"content\":{\"connectorIds\":[\"In1\"],\"side\":\"RIGHT\"},\"type\":\"ConnectorPlacement.EquallySpacedRectSide\",\"uuid\":\"a58e5db6-c2cf-479b-8575-444173ed86e1\"},{\"content\":{\"side\":\"TOP\"},\"type\":\"ConnectorPlacement.EquallySpacedRectSide\",\"uuid\":\"d8b1b400-2606-4583-b904-435fd1d8de03\"},{\"content\":{\"connectorIds\":[\"Out1\"],\"side\":\"BOTTOM\"},\"type\":\"ConnectorPlacement.EquallySpacedRectSide\",\"uuid\":\"4f056243-441b-49ed-b68a-00d3e0e63ccc\"}]},\"type\":\"ConnectorPlacement.EquallySpacedConnector\",\"uuid\":\"bef962c1-e5c2-4b6f-9336-41c558e2844c\"}],\"packageUris\":[\"http://schema.mathworks.com/mf0/Connector/R2020b\"],\"version\":\"1.0\"}"
  Bus Element Out1 : Outport  PortName=5V
  Bus Element Out3 : Outport  Port=2  PortName="Wattes  vlaues"
  Bus Element Out2 : Outport  Port=3  PortName=Trhemocouple[BMS-Digital]
  wires:
  Aux Battery/1(5V Raw) -> Fuse/1(5V Raw)
  Fuse/1("FuseProtected 5V ") -> E-Stop/1("FuseProtected 5V ")
  Thermocouple/1(Trhemocouple[BMS-Digital]) -> Bus Element Out2/1
  Power Meter/1(5V) -> Bus Element Out3/1
  E-Stop/1(E-Stop 5V) -> Thermocouple/1(5V), Power Meter/1(E-Stop 5V)
  connections:
  Thermocouple/RConn1 -- Aux Battery/RConn1

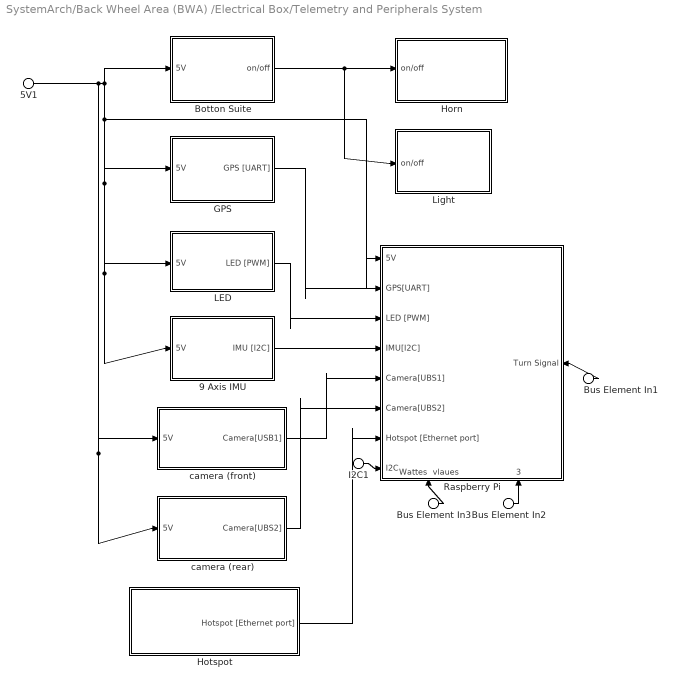
== system SystemArch/Back Wheel Area (BWA) /Electrical Box/Telemetry and Peripherals System ==
  Bus Element In3 : Inport  PortName="Wattes  vlaues"
  Bus Element In2 : Inport  Port=2  PortName=Trhemocouple[BMS-Digital]
  Bus Element In1 : Inport  Port=3  PortName=Turn Signal
  5V1 : Inport  Port=4  PortName=5V
  I2C1 : Inport  Port=5  PortName=I2C
  9 Axis IMU : Subsystem
      settings: PortSchema="{\"entries\":[{\"content\":{\"headerSize\":26,\"margin\":15,\"minimumSpacing\":25,\"sides\":[{\"content\":{\"connectorIds\":[\"In1\"]},\"type\":\"ConnectorPlacement.EquallySpacedRectSide\",\"uuid\":\"b908bc96-20ac-41af-bd35-1dc4c5c5d227\"},{\"content\":{\"connectorIds\":[\"Out1\"],\"side\":\"RIGHT\"},\"type\":\"ConnectorPlacement.EquallySpacedRectSide\",\"uuid\":\"a58e5db6-c2cf-479b-8575-444173ed86e1\"},{\"content\":{\"side\":\"TOP\"},\"type\":\"ConnectorPlacement.EquallySpacedRectSide\",\"uuid\":\"d8b1b400-2606-4583-b904-435fd1d8de03\"}]},\"type\":\"ConnectorPlacement.EquallySpacedConnector\",\"uuid\":\"bef962c1-e5c2-4b6f-9336-41c558e2844c\"}],\"packageUris\":[\"http://schema.mathworks.com/mf0/Connector/R2020b\"],\"version\":\"1.0\"}"
  Botton Suite : Subsystem
      settings: PortSchema="{\"entries\":[{\"content\":{\"headerSize\":26,\"margin\":15,\"minimumSpacing\":25,\"sides\":[{\"content\":{\"connectorIds\":[\"In1\"]},\"type\":\"ConnectorPlacement.EquallySpacedRectSide\",\"uuid\":\"e53759f5-b690-4877-b44a-d4eac11dffdb\"},{\"content\":{\"connectorIds\":[\"Out1\"],\"side\":\"RIGHT\"},\"type\":\"ConnectorPlacement.EquallySpacedRectSide\",\"uuid\":\"5814382e-6b7a-453f-be59-81d6220d088b\"},{\"content\":{\"side\":\"TOP\"},\"type\":\"ConnectorPlacement.EquallySpacedRectSide\",\"uuid\":\"b6b1eca2-b862-4844-b743-dac7054e5132\"}]},\"type\":\"ConnectorPlacement.EquallySpacedConnector\",\"uuid\":\"c2feee16-aff2-42ba-93bb-380b1af0aee9\"}],\"packageUris\":[\"http://schema.mathworks.com/mf0/Connector/R2020b\"],\"version\":\"1.0\"}"
  GPS : Subsystem
      settings: PortSchema="{\"entries\":[{\"content\":{\"headerSize\":26,\"margin\":15,\"minimumSpacing\":25,\"sides\":[{\"content\":{\"connectorIds\":[\"In1\"]},\"type\":\"ConnectorPlacement.EquallySpacedRectSide\",\"uuid\":\"b908bc96-20ac-41af-bd35-1dc4c5c5d227\"},{\"content\":{\"connectorIds\":[\"Out1\"],\"side\":\"RIGHT\"},\"type\":\"ConnectorPlacement.EquallySpacedRectSide\",\"uuid\":\"a58e5db6-c2cf-479b-8575-444173ed86e1\"},{\"content\":{\"side\":\"TOP\"},\"type\":\"ConnectorPlacement.EquallySpacedRectSide\",\"uuid\":\"d8b1b400-2606-4583-b904-435fd1d8de03\"}]},\"type\":\"ConnectorPlacement.EquallySpacedConnector\",\"uuid\":\"bef962c1-e5c2-4b6f-9336-41c558e2844c\"}],\"packageUris\":[\"http://schema.mathworks.com/mf0/Connector/R2020b\"],\"version\":\"1.0\"}"
  Horn : Subsystem
      settings: PortSchema="{\"entries\":[{\"content\":{\"headerSize\":26,\"margin\":15,\"minimumSpacing\":25,\"sides\":[{\"content\":{\"connectorIds\":[\"In1\"]},\"type\":\"ConnectorPlacement.EquallySpacedRectSide\",\"uuid\":\"b908bc96-20ac-41af-bd35-1dc4c5c5d227\"},{\"content\":{\"side\":\"RIGHT\"},\"type\":\"ConnectorPlacement.EquallySpacedRectSide\",\"uuid\":\"a58e5db6-c2cf-479b-8575-444173ed86e1\"},{\"content\":{\"side\":\"TOP\"},\"type\":\"ConnectorPlacement.EquallySpacedRectSide\",\"uuid\":\"d8b1b400-2606-4583-b904-435fd1d8de03\"}]},\"type\":\"ConnectorPlacement.EquallySpacedConnector\",\"uuid\":\"bef962c1-e5c2-4b6f-9336-41c558e2844c\"}],\"packageUris\":[\"http://schema.mathworks.com/mf0/Connector/R2020b\"],\"version\":\"1.0\"}"
  Hotspot : Subsystem
      settings: PortSchema="{\"entries\":[{\"content\":{\"headerSize\":26,\"margin\":15,\"minimumSpacing\":25,\"sides\":[{\"content\":{},\"type\":\"ConnectorPlacement.EquallySpacedRectSide\",\"uuid\":\"b908bc96-20ac-41af-bd35-1dc4c5c5d227\"},{\"content\":{\"connectorIds\":[\"Out1\"],\"side\":\"RIGHT\"},\"type\":\"ConnectorPlacement.EquallySpacedRectSide\",\"uuid\":\"a58e5db6-c2cf-479b-8575-444173ed86e1\"},{\"content\":{\"side\":\"TOP\"},\"type\":\"ConnectorPlacement.EquallySpacedRectSide\",\"uuid\":\"d8b1b400-2606-4583-b904-435fd1d8de03\"}]},\"type\":\"ConnectorPlacement.EquallySpacedConnector\",\"uuid\":\"bef962c1-e5c2-4b6f-9336-41c558e2844c\"}],\"packageUris\":[\"http://schema.mathworks.com/mf0/Connector/R2020b\"],\"version\":\"1.0\"}"
  LED : Subsystem
      settings: PortSchema="{\"entries\":[{\"content\":{\"headerSize\":26,\"margin\":15,\"minimumSpacing\":25,\"sides\":[{\"content\":{\"connectorIds\":[\"In1\"]},\"type\":\"ConnectorPlacement.EquallySpacedRectSide\",\"uuid\":\"b908bc96-20ac-41af-bd35-1dc4c5c5d227\"},{\"content\":{\"connectorIds\":[\"Out1\"],\"side\":\"RIGHT\"},\"type\":\"ConnectorPlacement.EquallySpacedRectSide\",\"uuid\":\"a58e5db6-c2cf-479b-8575-444173ed86e1\"},{\"content\":{\"side\":\"TOP\"},\"type\":\"ConnectorPlacement.EquallySpacedRectSide\",\"uuid\":\"d8b1b400-2606-4583-b904-435fd1d8de03\"}]},\"type\":\"ConnectorPlacement.EquallySpacedConnector\",\"uuid\":\"bef962c1-e5c2-4b6f-9336-41c558e2844c\"}],\"packageUris\":[\"http://schema.mathworks.com/mf0/Connector/R2020b\"],\"version\":\"1.0\"}"
  "Light " : Subsystem
      settings: PortSchema="{\"entries\":[{\"content\":{\"headerSize\":26,\"margin\":15,\"minimumSpacing\":25,\"sides\":[{\"content\":{\"connectorIds\":[\"In1\"]},\"type\":\"ConnectorPlacement.EquallySpacedRectSide\",\"uuid\":\"e53759f5-b690-4877-b44a-d4eac11dffdb\"},{\"content\":{\"side\":\"RIGHT\"},\"type\":\"ConnectorPlacement.EquallySpacedRectSide\",\"uuid\":\"5814382e-6b7a-453f-be59-81d6220d088b\"},{\"content\":{\"side\":\"TOP\"},\"type\":\"ConnectorPlacement.EquallySpacedRectSide\",\"uuid\":\"b6b1eca2-b862-4844-b743-dac7054e5132\"}]},\"type\":\"ConnectorPlacement.EquallySpacedConnector\",\"uuid\":\"c2feee16-aff2-42ba-93bb-380b1af0aee9\"}],\"packageUris\":[\"http://schema.mathworks.com/mf0/Connector/R2020b\"],\"version\":\"1.0\"}"
  Raspberry Pi : Subsystem
      settings: PortSchema="{\"entries\":[{\"content\":{\"headerSize\":26,\"margin\":15,\"minimumSpacing\":25,\"sides\":[{\"content\":{\"connectorIds\":[\"In4\",\"In5\",\"In6\",\"In7\",\"In8\",\"In9\",\"In10\",\"In11\"]},\"type\":\"ConnectorPlacement.EquallySpacedRectSide\",\"uuid\":\"b908bc96-20ac-41af-bd35-1dc4c5c5d227\"},{\"content\":{\"connectorIds\":[\"In1\"],\"side\":\"RIGHT\"},\"type\":\"ConnectorPlacement.EquallySpacedRectSide\",\"uuid\":\"a58e5db6-c2cf-479b-8575-444173ed86e1\"},{\"content\":{\"side\":\"TOP\"},\"type\":\"ConnectorPlacement.EquallySpacedRectSide\",\"uuid\":\"d8b1b400-2606-4583-b904-435fd1d8de03\"},{\"content\":{\"connectorIds\":[\"In2\",\"In3\"],\"side\":\"BOTTOM\"},\"type\":\"ConnectorPlacement.EquallySpacedRectSide\",\"uuid\":\"dd99c051-0a9a-410c-88eb-459a88827c2f\"}]},\"type\":\"ConnectorPlacement.EquallySpacedConnector\",\"uuid\":\"bef962c1-e5c2-4b6f-9336-41c558e2844c\"}],\"packageUris\":[\"http://schema.mathworks.com/mf0/Connector/R2020b\"],\"version\":\"1.0\"}"
  camera (front) : Subsystem
      settings: PortSchema="{\"entries\":[{\"content\":{\"headerSize\":26,\"margin\":15,\"minimumSpacing\":25,\"sides\":[{\"content\":{\"connectorIds\":[\"In1\"]},\"type\":\"ConnectorPlacement.EquallySpacedRectSide\",\"uuid\":\"b908bc96-20ac-41af-bd35-1dc4c5c5d227\"},{\"content\":{\"connectorIds\":[\"Out1\"],\"side\":\"RIGHT\"},\"type\":\"ConnectorPlacement.EquallySpacedRectSide\",\"uuid\":\"a58e5db6-c2cf-479b-8575-444173ed86e1\"},{\"content\":{\"side\":\"TOP\"},\"type\":\"ConnectorPlacement.EquallySpacedRectSide\",\"uuid\":\"d8b1b400-2606-4583-b904-435fd1d8de03\"}]},\"type\":\"ConnectorPlacement.EquallySpacedConnector\",\"uuid\":\"bef962c1-e5c2-4b6f-9336-41c558e2844c\"}],\"packageUris\":[\"http://schema.mathworks.com/mf0/Connector/R2020b\"],\"version\":\"1.0\"}"
  camera (rear) : Subsystem
      settings: PortSchema="{\"entries\":[{\"content\":{\"headerSize\":26,\"margin\":15,\"minimumSpacing\":25,\"sides\":[{\"content\":{\"connectorIds\":[\"In1\"]},\"type\":\"ConnectorPlacement.EquallySpacedRectSide\",\"uuid\":\"b908bc96-20ac-41af-bd35-1dc4c5c5d227\"},{\"content\":{\"connectorIds\":[\"Out1\"],\"side\":\"RIGHT\"},\"type\":\"ConnectorPlacement.EquallySpacedRectSide\",\"uuid\":\"a58e5db6-c2cf-479b-8575-444173ed86e1\"},{\"content\":{\"side\":\"TOP\"},\"type\":\"ConnectorPlacement.EquallySpacedRectSide\",\"uuid\":\"d8b1b400-2606-4583-b904-435fd1d8de03\"}]},\"type\":\"ConnectorPlacement.EquallySpacedConnector\",\"uuid\":\"bef962c1-e5c2-4b6f-9336-41c558e2844c\"}],\"packageUris\":[\"http://schema.mathworks.com/mf0/Connector/R2020b\"],\"version\":\"1.0\"}"
  wires:
  5V1/1 -> camera (front)/1(5V), camera (rear)/1(5V), 9 Axis IMU/1(5V), LED/1(5V), GPS/1(5V), Raspberry Pi/4(5V), Botton Suite/1(5V)
  9 Axis IMU/1(IMU [I2C]) -> Raspberry Pi/7(IMU[I2C])
  LED/1(LED [PWM]) -> Raspberry Pi/6(LED [PWM])
  camera (front)/1("Camera[USB1] ") -> Raspberry Pi/8("Camera[UBS1] ")
  Botton Suite/1(on/off) -> "Light "/1(on/off), Horn/1(on/off)
  Hotspot/1(Hotspot [Ethernet port]) -> Raspberry Pi/10(" Hotspot [Ethernet port]")
  GPS/1(GPS [UART]) -> Raspberry Pi/5(GPS[UART])
  camera (rear)/1(Camera[UBS2]) -> Raspberry Pi/9(Camera[UBS2])
  I2C1/1 -> Raspberry Pi/11(I2C)
  Bus Element In2/1 -> Raspberry Pi/3(Trhemocouple[BMS-Digital])
  Bus Element In3/1 -> Raspberry Pi/2("Wattes  vlaues ")
  Bus Element In1/1 -> Raspberry Pi/1(Turn Signal)
